simulink model "ass6_7_1"  (R2023a)
settings: Solver=VariableStepAuto  StartTime=0.0  StopTime=10.0  RelTol=1e-3
settings Model: Creator=Taniya Baral  LastModifiedBy=Taniya Baral

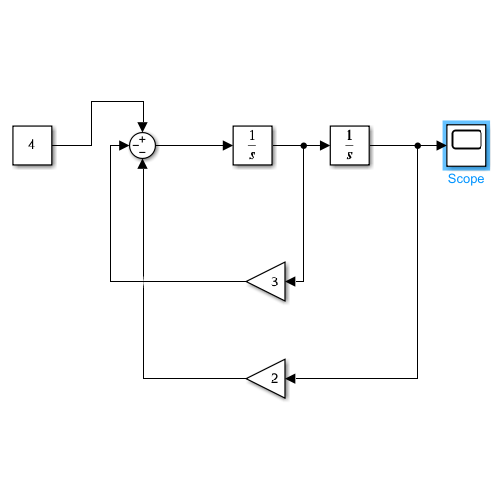
[thumbnail: Simulink's stored preview of the top-level diagram]
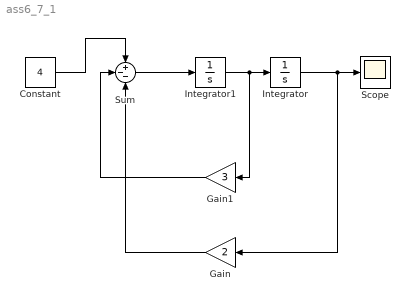
== system ass6_7_1 ==
  Constant : Constant  Value=4
  Gain : Gain  Gain=2
  Gain1 : Gain  Gain=3
  Integrator : Integrator
  Integrator1 : Integrator
  Scope : Scope
  Sum : Sum  Inputs=+--
  wires:
  Constant/1 -> Sum/1
  Sum/1 -> Integrator1/1
  Integrator1/1 -> Gain1/1, Integrator/1
  Integrator/1 -> Gain/1, Scope/1
  Gain1/1 -> Sum/2
  Gain/1 -> Sum/3
